simulink model "ES105A_StHlthSigNormn"  (R2013b)
settings: Solver=FixedStepDiscrete  SolverMode=SingleTasking  StartTime=0.0  StopTime=1  FixedStep=0.002  RelTol=1e-3
undefined symbols (not defined in the file): ARCHGLBPRM_FLOATZEROTHD_ULS_F32, CurrMeasCorrlnMaxErrCurr, CURRMOTSUMDIVBYZEROPROTNVAL_AMPR_F32, DIGTQDIVBYZEROPROTNVAL_HWNWTMTR_F32, DutyCycThermProtnDutyCycFildThd, EcuTMeasRngDiagcMax, EcuTMeasRngDiagcMin, EotLrngAuthyStrtLrn, FRICESTIMNDIVBYZEROPROTNVAL_HWNWTMTR_F32, HLTH0PERC_CNT_U08, HLTH100PERC_CNT_F32, HLTH100PERC_CNT_U08, HLTH50PERC_CNT_U08, HwTqCorrlnChATraSumSetFltThd, HwTqCorrlnChBTraSumSetFltThd, HWTQIDPTSIG_CNT_U08, MOTAG2MEAS_VALMAXERR_VOLTSQD_F32, MOTAG2MEAS_VALMINERR_VOLTSQD_F32, MOTAGCORRLN_MOTAGCORRLNERRTHD_MOTREVELEC_U0P16, MotDrvDiagcErrThd, MOTPOS2DIVBYZEROPROTNVAL2_VOLTSQD_F32, MOTPOS2DIVBYZEROPROTNVAL_VOLTSQD_F32, MOTPOSNERRDIVBYZEROPROTNVAL_MOTREV_U16, MOTPOSNERRZEROTHD_MOTREV_U0P16, NtcNr1, NtcSts1, PHAVLTGDIVBYZEROPROTNVAL_NANOSEC_F32, SigQlfr1, STHLTHSCAGFAC_CNT_F32, StHlthSigNormnAbsltMotPosDifStHlthDiagThd, StHlthSigNormnCurrMotSumStHlthDiagThd, StHlthSigNormnDigTqStHlthDiagThd, StHlthSigNormnDutyCycFltLimThd, StHlthSigNormnHiCtrlrT, StHlthSigNormnIdptSigStHlthSca, StHlthSigNormnLoCtrlrT, StHlthSigNormnMaxFricThd, StHlthSigNormnMinRackTrvlLim, StHlthSigNormnMotPosStHlthDiagThd, StHlthSigNormnMotVelCal, StHlthSigNormnPhaInfoStHlthDiagThd, StHlthSigNormnStHlthCorrlnErr, StHlthSigNormnStHlthCurrMotSum, StHlthSigNormnStHlthPhaInfo, StHlthSigNormnValMaxStHlthErr, StHlthSigNormnValMinStHlthErr, StHlthSigNormnWhlImbRejctnThd, SysGlbPrmMotPoleCnt, TSTHLTH0PERC_CNT_U08, u2, u3, u4, VLTGSTHLTH0PERC_CNT_U08
libraries: NxtrLim x39, simulink x33, NxtrAbslt x4
(part 4 of 10)

== system ES105A_StHlthSigNormn/StHlthSigNormn/UpdRawSig/Controller temperature/CtrlrTStHlth0Perc ==
  Action Port : ActionPort  ActionType=elseif
  Bitwise Operator : simulink/Logic and Bit Operations/Bitwise Operator  logicop=OR  UseBitMask=off  NumInputPorts=2  BitMask=bin2dec('11011001')  BitMaskRealWorld=Stored Integer
  Constant : Constant  Value=HLTH0PERC_CNT_U08  OutDataTypeStr=uint8
      settings: AttributesFormatString=%<OutDataTypeStr>
  Constant1 : Constant  OutDataTypeStr=uint8
      settings: AttributesFormatString=%<OutDataTypeStr>
  Constant2 : Constant  OutDataTypeStr=uint8
      settings: AttributesFormatString=%<OutDataTypeStr>
  CopyRight2 : Subsystem  Description=|  mask(Copyright Information){none=on}
      | Copyright info block.                                               
      |                                                                     
      | Place copyright information at the top of every subsystem in design.
      mask prompts: none "No parameters"
      mask help: Place copyright information at the top of every subsystem in design.
      mask Display:
      | NxtrConf = 'Nexteer Confidential';
      | 
      | sys = bdroot; %handle for the current model ("system")
      | first = get_param(sys,'Created');
      | first = first(end-3:end);  %year is last four digits
      | 
      | last = get_param(sys,'LastModifiedDate');
      | if isempty(last)
      |     last = datestr(now,'yyyy');
      | else
      |     last = last(end-3:end);
      | end
      | 
      | if strcmp(first,last)
      |     fprintf('%s -- Copyright %s Nexteer',NxtrConf,first)
      | else
      |     fprintf('%s -- %s%s- %s Nexteer',NxtrConf,char(169),first,last)
      | end
  Data Store Read : DataStoreRead  DataStoreName=EcuTRngIgnCyc
  Data Store Write : DataStoreWrite  DataStoreName=EcuTRngIgnCyc
  Shift Arithmetic : ArithShift  BitShiftNumber=LOTSTHLTH0PERC_CNT_U08  BitShiftDirection=Left
  Shift Arithmetic1 : ArithShift  BitShiftNumber=LOTSTHLTH0PERC_CNT_U08  BitShiftDirection=Left
  CtrlrTStHlth : Outport
  PrsntCtrlrTRng : Outport  Port=2
  wires:
  Shift Arithmetic1/1 -> PrsntCtrlrTRng/1
  Constant2/1 -> Shift Arithmetic1/1
  Bitwise Operator/1 -> Data Store Write/1
  Data Store Read/1 -> Bitwise Operator/1
  Shift Arithmetic/1 -> Bitwise Operator/2
  Constant1/1 -> Shift Arithmetic/1
  Constant/1 -> CtrlrTStHlth/1

== system ES105A_StHlthSigNormn/StHlthSigNormn/UpdRawSig/Controller temperature/CtrlrTStHlth0Perc1 ==
  Action Port : ActionPort  ActionType=else
  Bitwise Operator : simulink/Logic and Bit Operations/Bitwise Operator  logicop=OR  UseBitMask=off  NumInputPorts=2  BitMask=bin2dec('11011001')  BitMaskRealWorld=Stored Integer
  Constant : Constant  Value=HLTH0PERC_CNT_U08  OutDataTypeStr=uint8
      settings: AttributesFormatString=%<OutDataTypeStr>
  Constant1 : Constant  OutDataTypeStr=uint8
      settings: AttributesFormatString=%<OutDataTypeStr>
  Constant2 : Constant  OutDataTypeStr=uint8
      settings: AttributesFormatString=%<OutDataTypeStr>
  CopyRight2 : Subsystem  Description=|  mask(Copyright Information){none=on}
      | Copyright info block.                                               
      |                                                                     
      | Place copyright information at the top of every subsystem in design.
      mask prompts: none "No parameters"
      mask help: Place copyright information at the top of every subsystem in design.
      mask Display:
      | NxtrConf = 'Nexteer Confidential';
      | 
      | sys = bdroot; %handle for the current model ("system")
      | first = get_param(sys,'Created');
      | first = first(end-3:end);  %year is last four digits
      | 
      | last = get_param(sys,'LastModifiedDate');
      | if isempty(last)
      |     last = datestr(now,'yyyy');
      | else
      |     last = last(end-3:end);
      | end
      | 
      | if strcmp(first,last)
      |     fprintf('%s -- Copyright %s Nexteer',NxtrConf,first)
      | else
      |     fprintf('%s -- %s%s- %s Nexteer',NxtrConf,char(169),first,last)
      | end
  Data Store Read : DataStoreRead  DataStoreName=EcuTRngIgnCyc
  Data Store Write : DataStoreWrite  DataStoreName=EcuTRngIgnCyc
  Shift Arithmetic : ArithShift  BitShiftNumber=HITSTHLTH0PERC_CNT_U08  BitShiftDirection=Left
  Shift Arithmetic1 : ArithShift  BitShiftNumber=HITSTHLTH0PERC_CNT_U08  BitShiftDirection=Left
  CtrlrTStHlth : Outport
  PrsntCtrlrTRng : Outport  Port=2
  wires:
  Constant/1 -> CtrlrTStHlth/1
  Constant1/1 -> Shift Arithmetic/1
  Shift Arithmetic/1 -> Bitwise Operator/2
  Data Store Read/1 -> Bitwise Operator/1
  Bitwise Operator/1 -> Data Store Write/1
  Constant2/1 -> Shift Arithmetic1/1
  Shift Arithmetic1/1 -> PrsntCtrlrTRng/1

== system ES105A_StHlthSigNormn/StHlthSigNormn/UpdRawSig/Controller temperature/CtrlrTStHlth100Perc ==
  Action Port : ActionPort  ActionType=then
  Constant : Constant  Value=HLTH100PERC_CNT_U08  OutDataTypeStr=uint8
  Constant1 : Constant  Value=0  OutDataTypeStr=uint8
      settings: AttributesFormatString=%<OutDataTypeStr>
  CopyRight2 : Subsystem  Description=|  mask(Copyright Information){none=on}
      | Copyright info block.                                               
      |                                                                     
      | Place copyright information at the top of every subsystem in design.
      mask prompts: none "No parameters"
      mask help: Place copyright information at the top of every subsystem in design.
      mask Display:
      | NxtrConf = 'Nexteer Confidential';
      | 
      | sys = bdroot; %handle for the current model ("system")
      | first = get_param(sys,'Created');
      | first = first(end-3:end);  %year is last four digits
      | 
      | last = get_param(sys,'LastModifiedDate');
      | if isempty(last)
      |     last = datestr(now,'yyyy');
      | else
      |     last = last(end-3:end);
      | end
      | 
      | if strcmp(first,last)
      |     fprintf('%s -- Copyright %s Nexteer',NxtrConf,first)
      | else
      |     fprintf('%s -- %s%s- %s Nexteer',NxtrConf,char(169),first,last)
      | end
  CtrlrTStHlth : Outport
  PrsntCtrlrTRng : Outport  Port=2  InitialOutput=[0]
  wires:
  Constant/1 -> CtrlrTStHlth/1
  Constant1/1 -> PrsntCtrlrTRng/1

== system ES105A_StHlthSigNormn/StHlthSigNormn/UpdRawSig/Controller temperature/CtrlrTStHlth50Perc ==
  Action Port : ActionPort  ActionType=elseif
  Bitwise Operator : simulink/Logic and Bit Operations/Bitwise Operator  logicop=OR  UseBitMask=off  NumInputPorts=2  BitMask=bin2dec('11011001')  BitMaskRealWorld=Stored Integer
  Constant : Constant  Value=HLTH50PERC_CNT_U08  OutDataTypeStr=uint8
  Constant1 : Constant  OutDataTypeStr=uint8
      settings: AttributesFormatString=%<OutDataTypeStr>
  Constant2 : Constant  OutDataTypeStr=uint8
      settings: AttributesFormatString=%<OutDataTypeStr>
  CopyRight2 : Subsystem  Description=|  mask(Copyright Information){none=on}
      | Copyright info block.                                               
      |                                                                     
      | Place copyright information at the top of every subsystem in design.
      mask prompts: none "No parameters"
      mask help: Place copyright information at the top of every subsystem in design.
      mask Display:
      | NxtrConf = 'Nexteer Confidential';
      | 
      | sys = bdroot; %handle for the current model ("system")
      | first = get_param(sys,'Created');
      | first = first(end-3:end);  %year is last four digits
      | 
      | last = get_param(sys,'LastModifiedDate');
      | if isempty(last)
      |     last = datestr(now,'yyyy');
      | else
      |     last = last(end-3:end);
      | end
      | 
      | if strcmp(first,last)
      |     fprintf('%s -- Copyright %s Nexteer',NxtrConf,first)
      | else
      |     fprintf('%s -- %s%s- %s Nexteer',NxtrConf,char(169),first,last)
      | end
  Data Store Read : DataStoreRead  DataStoreName=EcuTRngIgnCyc
  Data Store Write : DataStoreWrite  DataStoreName=EcuTRngIgnCyc
  Shift Arithmetic : ArithShift  BitShiftNumber=LOTSTHLTH50PERC_CNT_U08  BitShiftDirection=Left
  Shift Arithmetic1 : ArithShift  BitShiftNumber=LOTSTHLTH50PERC_CNT_U08  BitShiftDirection=Left
  CtrlrTStHlth : Outport
  PrsntCtrlrTRng : Outport  Port=2
  wires:
  Constant/1 -> CtrlrTStHlth/1
  Constant1/1 -> Shift Arithmetic/1
  Shift Arithmetic/1 -> Bitwise Operator/2
  Data Store Read/1 -> Bitwise Operator/1
  Bitwise Operator/1 -> Data Store Write/1
  Constant2/1 -> Shift Arithmetic1/1
  Shift Arithmetic1/1 -> PrsntCtrlrTRng/1

== system ES105A_StHlthSigNormn/StHlthSigNormn/UpdRawSig/Controller temperature/CtrlrTStHlth50Perc1 ==
  Action Port : ActionPort  ActionType=elseif
  Bitwise Operator : simulink/Logic and Bit Operations/Bitwise Operator  logicop=OR  UseBitMask=off  NumInputPorts=2  BitMask=bin2dec('11011001')  BitMaskRealWorld=Stored Integer
  Constant : Constant  Value=HLTH50PERC_CNT_U08  OutDataTypeStr=uint8
      settings: AttributesFormatString=%<OutDataTypeStr>
  Constant1 : Constant  OutDataTypeStr=uint8
      settings: AttributesFormatString=%<OutDataTypeStr>
  Constant2 : Constant  OutDataTypeStr=uint8
      settings: AttributesFormatString=%<OutDataTypeStr>
  CopyRight2 : Subsystem  Description=|  mask(Copyright Information){none=on}
      | Copyright info block.                                               
      |                                                                     
      | Place copyright information at the top of every subsystem in design.
      mask prompts: none "No parameters"
      mask help: Place copyright information at the top of every subsystem in design.
      mask Display:
      | NxtrConf = 'Nexteer Confidential';
      | 
      | sys = bdroot; %handle for the current model ("system")
      | first = get_param(sys,'Created');
      | first = first(end-3:end);  %year is last four digits
      | 
      | last = get_param(sys,'LastModifiedDate');
      | if isempty(last)
      |     last = datestr(now,'yyyy');
      | else
      |     last = last(end-3:end);
      | end
      | 
      | if strcmp(first,last)
      |     fprintf('%s -- Copyright %s Nexteer',NxtrConf,first)
      | else
      |     fprintf('%s -- %s%s- %s Nexteer',NxtrConf,char(169),first,last)
      | end
  Data Store Read : DataStoreRead  DataStoreName=EcuTRngIgnCyc
  Data Store Write : DataStoreWrite  DataStoreName=EcuTRngIgnCyc
  Shift Arithmetic : ArithShift  BitShiftNumber=HITSTHLTH50PERC_CNT_U08  BitShiftDirection=Left
  Shift Arithmetic1 : ArithShift  BitShiftNumber=HITSTHLTH50PERC_CNT_U08  BitShiftDirection=Left
  CtrlrTStHlth : Outport
  PrsntCtrlrTRng : Outport  Port=2
  wires:
  Constant/1 -> CtrlrTStHlth/1
  Constant1/1 -> Shift Arithmetic/1
  Shift Arithmetic/1 -> Bitwise Operator/2
  Data Store Read/1 -> Bitwise Operator/1
  Bitwise Operator/1 -> Data Store Write/1
  Constant2/1 -> Shift Arithmetic1/1
  Shift Arithmetic1/1 -> PrsntCtrlrTRng/1

== system ES105A_StHlthSigNormn/StHlthSigNormn/UpdRawSig/Current Error/CopyRight2 ==

== system ES105A_StHlthSigNormn/StHlthSigNormn/UpdRawSig/Current Error/CurrMotSumABCStHlth Calc ==
  CurrMotSumABC : Inport
  Action Port : ActionPort  ActionType=case
  Constant : Constant  Value=StHlthSigNormnStHlthCurrMotSum
  CopyRight2 : Subsystem  Description=|  mask(Copyright Information){none=on}
      | Copyright info block.                                               
      |                                                                     
      | Place copyright information at the top of every subsystem in design.
      mask prompts: none "No parameters"
      mask help: Place copyright information at the top of every subsystem in design.
      mask Display:
      | NxtrConf = 'Nexteer Confidential';
      | 
      | sys = bdroot; %handle for the current model ("system")
      | first = get_param(sys,'Created');
      | first = first(end-3:end);  %year is last four digits
      | 
      | last = get_param(sys,'LastModifiedDate');
      | if isempty(last)
      |     last = datestr(now,'yyyy');
      | else
      |     last = last(end-3:end);
      | end
      | 
      | if strcmp(first,last)
      |     fprintf('%s -- Copyright %s Nexteer',NxtrConf,first)
      | else
      |     fprintf('%s -- %s%s- %s Nexteer',NxtrConf,char(169),first,last)
      | end
  If : If  IfExpression=u1
  If Action Subsystem : Subsystem  TreatAsAtomicUnit=on
  If Action Subsystem1 : Subsystem  TreatAsAtomicUnit=on
  LimStat_u2 : NxtrLim/LimStat_u08  LoLim=CurrMotSumABCStHlth.EngMin  HiLim=CurrMotSumABCStHlth.EngMax
      settings: AttributesFormatString=|
      | Low Limit: %<LoLim>
      | High Limit:%<HiLim>
  Merge : Merge
  Relational Operator : RelationalOperator  Operator=>  OutDataTypeStr=boolean
  CurrMotSumABCStHlth : Outport  InitialOutput=HLTH100PERC_CNT_U08
      settings: AttributesFormatString=Initial Output: %<InitialOutput>
  wires:
  CurrMotSumABC/1 -> [CurrMotSumABC], Relational Operator/1
  Constant/1 -> Relational Operator/2
  Relational Operator/1 -> If/1
  If/1 -> If Action Subsystem/Action
  If/2 -> If Action Subsystem1/Action
  [CurrMotSumABC] -> If Action Subsystem/1(CurrMotSumABC)
  If Action Subsystem/1(CurrMotSumABCStHlth) -> Merge/1
  If Action Subsystem1/1(CurrMotSumABCStHlth) -> Merge/2
  Merge/1 -> LimStat_u2/1
  LimStat_u2/1 -> CurrMotSumABCStHlth/1

== system ES105A_StHlthSigNormn/StHlthSigNormn/UpdRawSig/Current Error/CurrMotSumDEFStHlth Calc ==
  CurrMotSumDEF : Inport
  Action Port : ActionPort  ActionType=default
  Constant2 : Constant  Value=StHlthSigNormnStHlthCurrMotSum
  CopyRight2 : Subsystem  Description=|  mask(Copyright Information){none=on}
      | Copyright info block.                                               
      |                                                                     
      | Place copyright information at the top of every subsystem in design.
      mask prompts: none "No parameters"
      mask help: Place copyright information at the top of every subsystem in design.
      mask Display:
      | NxtrConf = 'Nexteer Confidential';
      | 
      | sys = bdroot; %handle for the current model ("system")
      | first = get_param(sys,'Created');
      | first = first(end-3:end);  %year is last four digits
      | 
      | last = get_param(sys,'LastModifiedDate');
      | if isempty(last)
      |     last = datestr(now,'yyyy');
      | else
      |     last = last(end-3:end);
      | end
      | 
      | if strcmp(first,last)
      |     fprintf('%s -- Copyright %s Nexteer',NxtrConf,first)
      | else
      |     fprintf('%s -- %s%s- %s Nexteer',NxtrConf,char(169),first,last)
      | end
  If Action Subsystem4 : Subsystem  TreatAsAtomicUnit=on
  If Action Subsystem5 : Subsystem  TreatAsAtomicUnit=on
  If2 : If  IfExpression=u1
  LimStat_u1 : NxtrLim/LimStat_u08  LoLim=CurrMotSumDEFStHlth.EngMin  HiLim=CurrMotSumDEFStHlth.EngMax
      settings: AttributesFormatString=|
      | Low Limit: %<LoLim>
      | High Limit:%<HiLim>
  Merge1 : Merge
  Relational Operator2 : RelationalOperator  Operator=>  OutDataTypeStr=boolean
  CurrMotSumDEFStHlth : Outport  InitialOutput=HLTH100PERC_CNT_U08
      settings: AttributesFormatString=Initial Output: %<InitialOutput>
  wires:
  CurrMotSumDEF/1 -> [CurrMotSumDEF], Relational Operator2/1
  Constant2/1 -> Relational Operator2/2
  Relational Operator2/1 -> If2/1
  If2/1 -> If Action Subsystem4/Action
  If2/2 -> If Action Subsystem5/Action
  [CurrMotSumDEF] -> If Action Subsystem4/1(CurrMotSumDEF)
  If Action Subsystem4/1(CurrMotSumDEFStHlth) -> Merge1/1
  If Action Subsystem5/1(CurrMotSumDEFStHlth) -> Merge1/2
  Merge1/1 -> LimStat_u1/1
  LimStat_u1/1 -> CurrMotSumDEFStHlth/1

== system ES105A_StHlthSigNormn/StHlthSigNormn/UpdRawSig/Current Error/CurrMotSumPhaStHlth ==
  NtcNr : Inport
  NtcStInfo : Inport  Port=2
  NtcSts : Inport  Port=3
  DebStep : Inport  Port=4
  SetNtcSts : Subsystem  RequirementInfo={} %GIDa_d68da11a_5186_43bd_ae15_b68d94f31a5a  TreatAsAtomicUnit=on
      settings: RTWSystemCode=Inline
  wires:
  NtcNr/1 -> SetNtcSts/1(NtcNr)  "NtcNr"
  NtcSts/1 -> SetNtcSts/3(NtcSts)
  DebStep/1 -> SetNtcSts/4(DebStep)
  NtcStInfo/1 -> SetNtcSts/2(NtcStInfo)

== system ES105A_StHlthSigNormn/StHlthSigNormn/UpdRawSig/Current Error/NTC Sts Calculation ==
  StHlthErr : Inport
  CopyRight2 : Subsystem  Description=|  mask(Copyright Information){none=on}
      | Copyright info block.                                               
      |                                                                     
      | Place copyright information at the top of every subsystem in design.
      mask prompts: none "No parameters"
      mask help: Place copyright information at the top of every subsystem in design.
      mask Display:
      | NxtrConf = 'Nexteer Confidential';
      | 
      | sys = bdroot; %handle for the current model ("system")
      | first = get_param(sys,'Created');
      | first = first(end-3:end);  %year is last four digits
      | 
      | last = get_param(sys,'LastModifiedDate');
      | if isempty(last)
      |     last = datestr(now,'yyyy');
      | else
      |     last = last(end-3:end);
      | end
      | 
      | if strcmp(first,last)
      |     fprintf('%s -- Copyright %s Nexteer',NxtrConf,first)
      | else
      |     fprintf('%s -- %s%s- %s Nexteer',NxtrConf,char(169),first,last)
      | end
  If : If  IfExpression=u1
  Merge : Merge
  NtcFaild : Subsystem  TreatAsAtomicUnit=on
  NtcPassd : Subsystem  TreatAsAtomicUnit=on
  NtcSts : Outport
  wires:
  StHlthErr/1 -> If/1
  If/1 -> NtcFaild/Action
  Merge/1 -> NtcSts/1
  NtcPassd/1(NtcPassd) -> Merge/2
  If/2 -> NtcPassd/Action
  NtcFaild/1(NtcFaild) -> Merge/1

== system ES105A_StHlthSigNormn/StHlthSigNormn/UpdRawSig/Default/CopyRight2 ==

== system ES105A_StHlthSigNormn/StHlthSigNormn/UpdRawSig/Digital Torque Sensor /CopyRight2 ==

== system ES105A_StHlthSigNormn/StHlthSigNormn/UpdRawSig/Digital Torque Sensor /DigTqIdptSigStHlth Calc ==
  HwTqIdptSig : Inport
  Action Port : ActionPort  ActionType=default
  Constant2 : Constant  Value=HWTQIDPTSIG_CNT_U08
  CopyRight2 : Subsystem  Description=|  mask(Copyright Information){none=on}
      | Copyright info block.                                               
      |                                                                     
      | Place copyright information at the top of every subsystem in design.
      mask prompts: none "No parameters"
      mask help: Place copyright information at the top of every subsystem in design.
      mask Display:
      | NxtrConf = 'Nexteer Confidential';
      | 
      | sys = bdroot; %handle for the current model ("system")
      | first = get_param(sys,'Created');
      | first = first(end-3:end);  %year is last four digits
      | 
      | last = get_param(sys,'LastModifiedDate');
      | if isempty(last)
      |     last = datestr(now,'yyyy');
      | else
      |     last = last(end-3:end);
      | end
      | 
      | if strcmp(first,last)
      |     fprintf('%s -- Copyright %s Nexteer',NxtrConf,first)
      | else
      |     fprintf('%s -- %s%s- %s Nexteer',NxtrConf,char(169),first,last)
      | end
  If Action Subsystem4 : Subsystem  TreatAsAtomicUnit=on
  If Action Subsystem5 : Subsystem  TreatAsAtomicUnit=on
  If2 : If  IfExpression=u1
  LimStat_u2 : NxtrLim/LimStat_u08  LoLim=DigTqIdptSigStHlth.EngMin  HiLim=DigTqIdptSigStHlth.EngMax
      settings: AttributesFormatString=|
      | Low Limit: %<LoLim>
      | High Limit:%<HiLim>
  Merge2 : Merge
  Relational Operator2 : RelationalOperator  Operator===  OutDataTypeStr=boolean
  " DigTqIdptSigStHlth" : Outport  InitialOutput=HLTH100PERC_CNT_U08
      settings: AttributesFormatString=Initial Output: %<InitialOutput>
  wires:
  Relational Operator2/1 -> If2/1
  If2/1 -> If Action Subsystem4/Action
  If2/2 -> If Action Subsystem5/Action
  HwTqIdptSig/1 -> If Action Subsystem5/1(HwTqIdptSig), Relational Operator2/1
  If Action Subsystem4/1(DigTqIdptSigStHlth) -> Merge2/1
  Merge2/1 -> LimStat_u2/1
  Constant2/1 -> Relational Operator2/2
  If Action Subsystem5/1(DigTqIdptSigStHlth) -> Merge2/2
  LimStat_u2/1 -> " DigTqIdptSigStHlth"/1

== system ES105A_StHlthSigNormn/StHlthSigNormn/UpdRawSig/Digital Torque Sensor /DigTqSnsrAStHlth Calc ==
  HwTqChACorrlnTraErr : Inport
  Action Port : ActionPort  ActionType=case
  Abslt_f32_f32 : NxtrAbslt/Abslt_f32_f32  SFunctionSpec=single y1 = Abslt_f32_f32(single u1)
      settings: AttributesFormatString=%<Name>
  Constant : Constant  Value=HwTqCorrlnChATraSumSetFltThd
  CopyRight2 : Subsystem  Description=|  mask(Copyright Information){none=on}
      | Copyright info block.                                               
      |                                                                     
      | Place copyright information at the top of every subsystem in design.
      mask prompts: none "No parameters"
      mask help: Place copyright information at the top of every subsystem in design.
      mask Display:
      | NxtrConf = 'Nexteer Confidential';
      | 
      | sys = bdroot; %handle for the current model ("system")
      | first = get_param(sys,'Created');
      | first = first(end-3:end);  %year is last four digits
      | 
      | last = get_param(sys,'LastModifiedDate');
      | if isempty(last)
      |     last = datestr(now,'yyyy');
      | else
      |     last = last(end-3:end);
      | end
      | 
      | if strcmp(first,last)
      |     fprintf('%s -- Copyright %s Nexteer',NxtrConf,first)
      | else
      |     fprintf('%s -- %s%s- %s Nexteer',NxtrConf,char(169),first,last)
      | end
  If : If  IfExpression=u1
  If Action Subsystem : Subsystem  TreatAsAtomicUnit=on
  If Action Subsystem1 : Subsystem  TreatAsAtomicUnit=on
  LimStat_u08 : NxtrLim/LimStat_u08  LoLim=DigTqSnsrAStHlth.EngMin  HiLim=DigTqSnsrAStHlth.EngMax
      settings: AttributesFormatString=|
      | Low Limit: %<LoLim>
      | High Limit:%<HiLim>
  Merge : Merge
  Relational Operator : RelationalOperator  Operator=>  OutDataTypeStr=boolean
  DigTqSnsrAStHlth : Outport  InitialOutput=HLTH100PERC_CNT_U08
      settings: AttributesFormatString=Initial Output: %<InitialOutput>
  wires:
  Merge/1 -> LimStat_u08/1
  Abslt_f32_f32/1 -> Relational Operator/1
  Constant/1 -> Relational Operator/2
  Relational Operator/1 -> If/1
  If/1 -> If Action Subsystem/Action
  If/2 -> If Action Subsystem1/Action
  HwTqChACorrlnTraErr/1 -> Abslt_f32_f32/1, If Action Subsystem1/1(HwTqChACorrlnTraErr)
  If Action Subsystem/1(DigTqSnsrAStHlth) -> Merge/1
  If Action Subsystem1/1(DigTqSnsrAStHlth) -> Merge/2
  LimStat_u08/1 -> DigTqSnsrAStHlth/1

== system ES105A_StHlthSigNormn/StHlthSigNormn/UpdRawSig/Digital Torque Sensor /DigTqSnsrBStHlth Calc ==
  HwTqChBCorrlnTraErr : Inport
  Action Port : ActionPort  ActionType=case
  Abslt_f32_f1 : NxtrAbslt/Abslt_f32_f32  SFunctionSpec=single y1 = Abslt_f32_f32(single u1)
      settings: AttributesFormatString=%<Name>
  Constant1 : Constant  Value=HwTqCorrlnChBTraSumSetFltThd
  CopyRight2 : Subsystem  Description=|  mask(Copyright Information){none=on}
      | Copyright info block.                                               
      |                                                                     
      | Place copyright information at the top of every subsystem in design.
      mask prompts: none "No parameters"
      mask help: Place copyright information at the top of every subsystem in design.
      mask Display:
      | NxtrConf = 'Nexteer Confidential';
      | 
      | sys = bdroot; %handle for the current model ("system")
      | first = get_param(sys,'Created');
      | first = first(end-3:end);  %year is last four digits
      | 
      | last = get_param(sys,'LastModifiedDate');
      | if isempty(last)
      |     last = datestr(now,'yyyy');
      | else
      |     last = last(end-3:end);
      | end
      | 
      | if strcmp(first,last)
      |     fprintf('%s -- Copyright %s Nexteer',NxtrConf,first)
      | else
      |     fprintf('%s -- %s%s- %s Nexteer',NxtrConf,char(169),first,last)
      | end
  If Action Subsystem2 : Subsystem  TreatAsAtomicUnit=on
  If Action Subsystem3 : Subsystem  TreatAsAtomicUnit=on
  If1 : If  IfExpression=u1
  LimStat_u1 : NxtrLim/LimStat_u08  LoLim=DigTqSnsrBStHlth.EngMin  HiLim=DigTqSnsrBStHlth.EngMax
      settings: AttributesFormatString=|
      | Low Limit: %<LoLim>
      | High Limit:%<HiLim>
  Merge1 : Merge
  Relational Operator1 : RelationalOperator  Operator=>  OutDataTypeStr=boolean
  DigTqSnsrBStHlth : Outport  InitialOutput=HLTH100PERC_CNT_U08
      settings: AttributesFormatString=Initial Output: %<InitialOutput>
  wires:
  Merge1/1 -> LimStat_u1/1
  Abslt_f32_f1/1 -> Relational Operator1/1
  Constant1/1 -> Relational Operator1/2
  Relational Operator1/1 -> If1/1
  If1/1 -> If Action Subsystem2/Action
  If1/2 -> If Action Subsystem3/Action
  HwTqChBCorrlnTraErr/1 -> Abslt_f32_f1/1, If Action Subsystem3/1(HwTqChBCorrlnTraErr)
  If Action Subsystem2/1(DigTqSnsrBStHlth) -> Merge1/1
  If Action Subsystem3/1(DigTqSnsrBStHlth) -> Merge1/2
  LimStat_u1/1 -> DigTqSnsrBStHlth/1

== system ES105A_StHlthSigNormn/StHlthSigNormn/UpdRawSig/Digital Torque Sensor /DigTqSnsrPhaStHlth ==
  NtcNr : Inport
  NtcStInfo : Inport  Port=2
  NtcSts : Inport  Port=3
  DebStep : Inport  Port=4
  SetNtcSts : Subsystem  RequirementInfo={} %GIDa_2e8106b4_b705_4f70_a166_c375d4b30e66  TreatAsAtomicUnit=on
      settings: RTWSystemCode=Inline
  wires:
  NtcNr/1 -> SetNtcSts/1(NtcNr)  "NtcNr"
  NtcSts/1 -> SetNtcSts/3(NtcSts)
  DebStep/1 -> SetNtcSts/4(DebStep)
  NtcStInfo/1 -> SetNtcSts/2(NtcStInfo)

== system ES105A_StHlthSigNormn/StHlthSigNormn/UpdRawSig/Digital Torque Sensor /NTC Sts Calculation ==
  StHlthErr : Inport
  CopyRight2 : Subsystem  Description=|  mask(Copyright Information){none=on}
      | Copyright info block.                                               
      |                                                                     
      | Place copyright information at the top of every subsystem in design.
      mask prompts: none "No parameters"
      mask help: Place copyright information at the top of every subsystem in design.
      mask Display:
      | NxtrConf = 'Nexteer Confidential';
      | 
      | sys = bdroot; %handle for the current model ("system")
      | first = get_param(sys,'Created');
      | first = first(end-3:end);  %year is last four digits
      | 
      | last = get_param(sys,'LastModifiedDate');
      | if isempty(last)
      |     last = datestr(now,'yyyy');
      | else
      |     last = last(end-3:end);
      | end
      | 
      | if strcmp(first,last)
      |     fprintf('%s -- Copyright %s Nexteer',NxtrConf,first)
      | else
      |     fprintf('%s -- %s%s- %s Nexteer',NxtrConf,char(169),first,last)
      | end
  If : If  IfExpression=u1
  Merge : Merge
  NtcFaild : Subsystem  TreatAsAtomicUnit=on
  NtcPassd : Subsystem  TreatAsAtomicUnit=on
  NtcSts : Outport
  wires:
  StHlthErr/1 -> If/1
  If/1 -> NtcFaild/Action
  Merge/1 -> NtcSts/1
  NtcPassd/1(NtcPassd) -> Merge/2
  If/2 -> NtcPassd/Action
  NtcFaild/1(NtcFaild) -> Merge/1

== system ES105A_StHlthSigNormn/StHlthSigNormn/UpdRawSig/Duty Cycle Exceeded/CopyRight2 ==

== system ES105A_StHlthSigNormn/StHlthSigNormn/UpdRawSig/Duty Cycle Exceeded/If Action Subsystem ==
  Action Port : ActionPort  ActionType=then
  Constant : Constant  Value=HLTH0PERC_CNT_U08
  CopyRight2 : Subsystem  Description=|  mask(Copyright Information){none=on}
      | Copyright info block.                                               
      |                                                                     
      | Place copyright information at the top of every subsystem in design.
      mask prompts: none "No parameters"
      mask help: Place copyright information at the top of every subsystem in design.
      mask Display:
      | NxtrConf = 'Nexteer Confidential';
      | 
      | sys = bdroot; %handle for the current model ("system")
      | first = get_param(sys,'Created');
      | first = first(end-3:end);  %year is last four digits
      | 
      | last = get_param(sys,'LastModifiedDate');
      | if isempty(last)
      |     last = datestr(now,'yyyy');
      | else
      |     last = last(end-3:end);
      | end
      | 
      | if strcmp(first,last)
      |     fprintf('%s -- Copyright %s Nexteer',NxtrConf,first)
      | else
      |     fprintf('%s -- %s%s- %s Nexteer',NxtrConf,char(169),first,last)
      | end
  DutyCycStHlth : Outport
  wires:
  Constant/1 -> DutyCycStHlth/1

== system ES105A_StHlthSigNormn/StHlthSigNormn/UpdRawSig/Duty Cycle Exceeded/If Action Subsystem1 ==
  Action Port : ActionPort  ActionType=elseif
  Constant : Constant  Value=HLTH50PERC_CNT_U08
  CopyRight2 : Subsystem  Description=|  mask(Copyright Information){none=on}
      | Copyright info block.                                               
      |                                                                     
      | Place copyright information at the top of every subsystem in design.
      mask prompts: none "No parameters"
      mask help: Place copyright information at the top of every subsystem in design.
      mask Display:
      | NxtrConf = 'Nexteer Confidential';
      | 
      | sys = bdroot; %handle for the current model ("system")
      | first = get_param(sys,'Created');
      | first = first(end-3:end);  %year is last four digits
      | 
      | last = get_param(sys,'LastModifiedDate');
      | if isempty(last)
      |     last = datestr(now,'yyyy');
      | else
      |     last = last(end-3:end);
      | end
      | 
      | if strcmp(first,last)
      |     fprintf('%s -- Copyright %s Nexteer',NxtrConf,first)
      | else
      |     fprintf('%s -- %s%s- %s Nexteer',NxtrConf,char(169),first,last)
      | end
  DutyCycStHlth : Outport
  wires:
  Constant/1 -> DutyCycStHlth/1

== system ES105A_StHlthSigNormn/StHlthSigNormn/UpdRawSig/Duty Cycle Exceeded/If Action Subsystem2 ==
  Action Port : ActionPort  ActionType=else
  Constant : Constant  Value=HLTH100PERC_CNT_U08
  CopyRight2 : Subsystem  Description=|  mask(Copyright Information){none=on}
      | Copyright info block.                                               
      |                                                                     
      | Place copyright information at the top of every subsystem in design.
      mask prompts: none "No parameters"
      mask help: Place copyright information at the top of every subsystem in design.
      mask Display:
      | NxtrConf = 'Nexteer Confidential';
      | 
      | sys = bdroot; %handle for the current model ("system")
      | first = get_param(sys,'Created');
      | first = first(end-3:end);  %year is last four digits
      | 
      | last = get_param(sys,'LastModifiedDate');
      | if isempty(last)
      |     last = datestr(now,'yyyy');
      | else
      |     last = last(end-3:end);
      | end
      | 
      | if strcmp(first,last)
      |     fprintf('%s -- Copyright %s Nexteer',NxtrConf,first)
      | else
      |     fprintf('%s -- %s%s- %s Nexteer',NxtrConf,char(169),first,last)
      | end
  DutyCycStHlth : Outport
  wires:
  Constant/1 -> DutyCycStHlth/1

== system ES105A_StHlthSigNormn/StHlthSigNormn/UpdRawSig/Friction Estimation/CopyRight2 ==

== system ES105A_StHlthSigNormn/StHlthSigNormn/UpdRawSig/Friction Estimation/If Action Subsystem3 ==
  Action Port : ActionPort  ActionType=else
  Constant : Constant  Value=HLTH0PERC_CNT_U08
  CopyRight2 : Subsystem  Description=|  mask(Copyright Information){none=on}
      | Copyright info block.                                               
      |                                                                     
      | Place copyright information at the top of every subsystem in design.
      mask prompts: none "No parameters"
      mask help: Place copyright information at the top of every subsystem in design.
      mask Display:
      | NxtrConf = 'Nexteer Confidential';
      | 
      | sys = bdroot; %handle for the current model ("system")
      | first = get_param(sys,'Created');
      | first = first(end-3:end);  %year is last four digits
      | 
      | last = get_param(sys,'LastModifiedDate');
      | if isempty(last)
      |     last = datestr(now,'yyyy');
      | else
      |     last = last(end-3:end);
      | end
      | 
      | if strcmp(first,last)
      |     fprintf('%s -- Copyright %s Nexteer',NxtrConf,first)
      | else
      |     fprintf('%s -- %s%s- %s Nexteer',NxtrConf,char(169),first,last)
      | end
  FricEstStHlth : Outport
  wires:
  Constant/1 -> FricEstStHlth/1

== system ES105A_StHlthSigNormn/StHlthSigNormn/UpdRawSig/Friction Estimation/If Action Subsystem4 ==
  MaxLrndFric : Inport
  EOLFric : Inport  Port=2
  Action Port : ActionPort  ActionType=then
  Abs : Abs
  Add : Sum  Inputs=+-
  Add1 : Sum  Inputs=+-
  Constant1 : Constant  OutDataTypeStr=single
      settings: AttributesFormatString=%<OutDataTypeStr>
  Constant4 : Constant  Value=HLTH100PERC_CNT_F32
  CopyRight2 : Subsystem  Description=|  mask(Copyright Information){none=on}
      | Copyright info block.                                               
      |                                                                     
      | Place copyright information at the top of every subsystem in design.
      mask prompts: none "No parameters"
      mask help: Place copyright information at the top of every subsystem in design.
      mask Display:
      | NxtrConf = 'Nexteer Confidential';
      | 
      | sys = bdroot; %handle for the current model ("system")
      | first = get_param(sys,'Created');
      | first = first(end-3:end);  %year is last four digits
      | 
      | last = get_param(sys,'LastModifiedDate');
      | if isempty(last)
      |     last = datestr(now,'yyyy');
      | else
      |     last = last(end-3:end);
      | end
      | 
      | if strcmp(first,last)
      |     fprintf('%s -- Copyright %s Nexteer',NxtrConf,first)
      | else
      |     fprintf('%s -- %s%s- %s Nexteer',NxtrConf,char(169),first,last)
      | end
  Data Type Conversion : DataTypeConversion  OutDataTypeStr=uint8
  Divide : Product  Inputs=*/
  Divide by Zero Protection for Cal : Subsystem
  LimStat_f32 : NxtrLim/LimStat_f32  LoLim=FRICESTSTHLTHLOLI_CNT_F32  HiLim=FRICESTSTHLTHHILI_CNT_F32
      settings: AttributesFormatString=|
      | Low Limit: %<LoLim>
      | High Limit:%<HiLim>
  Product : Product
  FricEstStHlth : Outport
  wires:
  Constant1/1 -> Add/1
  Constant4/1 -> Product/2
  LimStat_f32/1 -> Data Type Conversion/1
  Data Type Conversion/1 -> FricEstStHlth/1
  Divide by Zero Protection for Cal/1(FricEstDelta) -> Divide/2
  MaxLrndFric/1 -> Add1/1
  Product/1 -> LimStat_f32/1
  Add/1 -> Product/1
  EOLFric/1 -> Add1/2, [EOLFric]
  Divide/1 -> Add/2
  Add1/1 -> Abs/1
  Abs/1 -> Divide/1
  [EOLFric] -> Divide by Zero Protection for Cal/1(EOLFric)

== system ES105A_StHlthSigNormn/StHlthSigNormn/UpdRawSig/Motor Position 2 /CopyRight2 ==

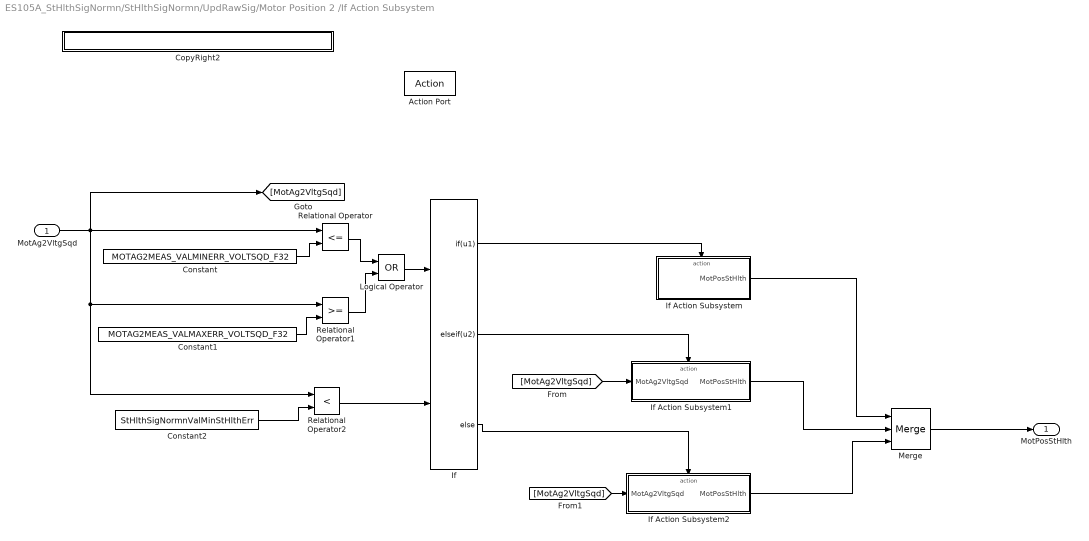
== system ES105A_StHlthSigNormn/StHlthSigNormn/UpdRawSig/Motor Position 2 /If Action Subsystem ==
  MotAg2VltgSqd : Inport
  Action Port : ActionPort  ActionType=then
  Constant : Constant  Value=MOTAG2MEAS_VALMINERR_VOLTSQD_F32
  Constant1 : Constant  Value=MOTAG2MEAS_VALMAXERR_VOLTSQD_F32
  Constant2 : Constant  Value=StHlthSigNormnValMinStHlthErr
  CopyRight2 : Subsystem  Description=|  mask(Copyright Information){none=on}
      | Copyright info block.                                               
      |                                                                     
      | Place copyright information at the top of every subsystem in design.
      mask prompts: none "No parameters"
      mask help: Place copyright information at the top of every subsystem in design.
      mask Display:
      | NxtrConf = 'Nexteer Confidential';
      | 
      | sys = bdroot; %handle for the current model ("system")
      | first = get_param(sys,'Created');
      | first = first(end-3:end);  %year is last four digits
      | 
      | last = get_param(sys,'LastModifiedDate');
      | if isempty(last)
      |     last = datestr(now,'yyyy');
      | else
      |     last = last(end-3:end);
      | end
      | 
      | if strcmp(first,last)
      |     fprintf('%s -- Copyright %s Nexteer',NxtrConf,first)
      | else
      |     fprintf('%s -- %s%s- %s Nexteer',NxtrConf,char(169),first,last)
      | end
  If : If  NumInputs=2  IfExpression=u1  ElseIfExpressions=u2
  If Action Subsystem : Subsystem  TreatAsAtomicUnit=on
  If Action Subsystem1 : Subsystem  TreatAsAtomicUnit=on
  If Action Subsystem2 : Subsystem  TreatAsAtomicUnit=on
  Logical Operator : Logic  Operator=OR  AllPortsSameDT=off  OutDataTypeStr=boolean
  Merge : Merge  Inputs=3
  Relational Operator : RelationalOperator  Operator=<=  OutDataTypeStr=boolean
  Relational Operator1 : RelationalOperator  OutDataTypeStr=boolean
  Relational Operator2 : RelationalOperator  Operator=<  OutDataTypeStr=boolean
  MotPosStHlth : Outport
  wires:
  Constant/1 -> Relational Operator/2
  MotAg2VltgSqd/1 -> Relational Operator/1, [MotAg2VltgSqd], Relational Operator1/1, Relational Operator2/1
  Constant1/1 -> Relational Operator1/2
  Relational Operator/1 -> Logical Operator/1
  Relational Operator1/1 -> Logical Operator/2
  Logical Operator/1 -> If/1
  If/1 -> If Action Subsystem/Action
  Constant2/1 -> Relational Operator2/2
  Relational Operator2/1 -> If/2
  If/2 -> If Action Subsystem1/Action
  If/3 -> If Action Subsystem2/Action
  [MotAg2VltgSqd] -> If Action Subsystem1/1(MotAg2VltgSqd)
  [MotAg2VltgSqd] -> If Action Subsystem2/1(MotAg2VltgSqd)
  If Action Subsystem/1(MotPosStHlth) -> Merge/1
  Merge/1 -> MotPosStHlth/1
  If Action Subsystem2/1(MotPosStHlth) -> Merge/3
  If Action Subsystem1/1(MotPosStHlth) -> Merge/2

== system ES105A_StHlthSigNormn/StHlthSigNormn/UpdRawSig/Motor Position 2 /If Action Subsystem1 ==
  Action Port : ActionPort  ActionType=else
  Constant : Constant  Value=HLTH100PERC_CNT_U08
  CopyRight2 : Subsystem  Description=|  mask(Copyright Information){none=on}
      | Copyright info block.                                               
      |                                                                     
      | Place copyright information at the top of every subsystem in design.
      mask prompts: none "No parameters"
      mask help: Place copyright information at the top of every subsystem in design.
      mask Display:
      | NxtrConf = 'Nexteer Confidential';
      | 
      | sys = bdroot; %handle for the current model ("system")
      | first = get_param(sys,'Created');
      | first = first(end-3:end);  %year is last four digits
      | 
      | last = get_param(sys,'LastModifiedDate');
      | if isempty(last)
      |     last = datestr(now,'yyyy');
      | else
      |     last = last(end-3:end);
      | end
      | 
      | if strcmp(first,last)
      |     fprintf('%s -- Copyright %s Nexteer',NxtrConf,first)
      | else
      |     fprintf('%s -- %s%s- %s Nexteer',NxtrConf,char(169),first,last)
      | end
  MotPosStHlth : Outport
  wires:
  Constant/1 -> MotPosStHlth/1

== system ES105A_StHlthSigNormn/StHlthSigNormn/UpdRawSig/Motor Position 2 /NTC Sts Calculation ==
  StHlthErr : Inport
  CopyRight2 : Subsystem  Description=|  mask(Copyright Information){none=on}
      | Copyright info block.                                               
      |                                                                     
      | Place copyright information at the top of every subsystem in design.
      mask prompts: none "No parameters"
      mask help: Place copyright information at the top of every subsystem in design.
      mask Display:
      | NxtrConf = 'Nexteer Confidential';
      | 
      | sys = bdroot; %handle for the current model ("system")
      | first = get_param(sys,'Created');
      | first = first(end-3:end);  %year is last four digits
      | 
      | last = get_param(sys,'LastModifiedDate');
      | if isempty(last)
      |     last = datestr(now,'yyyy');
      | else
      |     last = last(end-3:end);
      | end
      | 
      | if strcmp(first,last)
      |     fprintf('%s -- Copyright %s Nexteer',NxtrConf,first)
      | else
      |     fprintf('%s -- %s%s- %s Nexteer',NxtrConf,char(169),first,last)
      | end
  If : If  IfExpression=u1
  Merge : Merge
  NtcFaild : Subsystem  TreatAsAtomicUnit=on
  NtcPassd : Subsystem  TreatAsAtomicUnit=on
  NtcSts : Outport
  wires:
  StHlthErr/1 -> If/1
  If/1 -> NtcFaild/Action
  Merge/1 -> NtcSts/1
  NtcPassd/1(NtcPassd) -> Merge/2
  If/2 -> NtcPassd/Action
  NtcFaild/1(NtcFaild) -> Merge/1

== system ES105A_StHlthSigNormn/StHlthSigNormn/UpdRawSig/Motor Position 2 /NtcMotPosStHlth ==
  NtcNr : Inport
  NtcStInfo : Inport  Port=2
  NtcSts : Inport  Port=3
  DebStep : Inport  Port=4
  SetNtcSts : Subsystem  RequirementInfo={} %GIDa_e15acc41_e270_4229_a20a_2a1d705a48ba  TreatAsAtomicUnit=on
      settings: RTWSystemCode=Inline
  wires:
  NtcNr/1 -> SetNtcSts/1(NtcNr)  "NtcNr"
  NtcSts/1 -> SetNtcSts/3(NtcSts)
  DebStep/1 -> SetNtcSts/4(DebStep)
  NtcStInfo/1 -> SetNtcSts/2(NtcStInfo)

== system ES105A_StHlthSigNormn/StHlthSigNormn/UpdRawSig/Motor Position Error /AbsltMotPosABDifStHlth Calc ==
  MotAgABErrTerm : Inport
  Action Port : ActionPort  ActionType=case
  Constant : Constant  Value=StHlthSigNormnStHlthCorrlnErr
  CopyRight2 : Subsystem  Description=|  mask(Copyright Information){none=on}
      | Copyright info block.                                               
      |                                                                     
      | Place copyright information at the top of every subsystem in design.
      mask prompts: none "No parameters"
      mask help: Place copyright information at the top of every subsystem in design.
      mask Display:
      | NxtrConf = 'Nexteer Confidential';
      | 
      | sys = bdroot; %handle for the current model ("system")
      | first = get_param(sys,'Created');
      | first = first(end-3:end);  %year is last four digits
      | 
      | last = get_param(sys,'LastModifiedDate');
      | if isempty(last)
      |     last = datestr(now,'yyyy');
      | else
      |     last = last(end-3:end);
      | end
      | 
      | if strcmp(first,last)
      |     fprintf('%s -- Copyright %s Nexteer',NxtrConf,first)
      | else
      |     fprintf('%s -- %s%s- %s Nexteer',NxtrConf,char(169),first,last)
      | end
  If : If  IfExpression=u1
  If Action Subsystem : Subsystem  TreatAsAtomicUnit=on
  If Action Subsystem1 : Subsystem  TreatAsAtomicUnit=on
  LimStat_u2 : NxtrLim/LimStat_u08  LoLim=AbsltMotPosABDifStHlth.EngMin  HiLim=AbsltMotPosABDifStHlth.EngMax
      settings: AttributesFormatString=|
      | Low Limit: %<LoLim>
      | High Limit:%<HiLim>
  Merge : Merge
  Relational Operator : RelationalOperator  Operator=>  OutDataTypeStr=boolean
  AbsltMotPosABDifStHlth : Outport  InitialOutput=HLTH100PERC_CNT_U08
      settings: AttributesFormatString=Initial Output: %<InitialOutput>
  wires:
  MotAgABErrTerm/1 -> [MotAgABErrTerm], Relational Operator/1
  Constant/1 -> Relational Operator/2
  Relational Operator/1 -> If/1
  If/1 -> If Action Subsystem/Action
  If/2 -> If Action Subsystem1/Action
  [MotAgABErrTerm] -> If Action Subsystem/1(MotAgABErrTerm)
  If Action Subsystem/1(AbsltMotPosABDiffStHlth) -> Merge/1
  If Action Subsystem1/1(AbsltMotPosABDiffStHlth) -> Merge/2
  Merge/1 -> LimStat_u2/1
  LimStat_u2/1 -> AbsltMotPosABDifStHlth/1

== system ES105A_StHlthSigNormn/StHlthSigNormn/UpdRawSig/Motor Position Error /AbsltMotPosACDifStHlth Calc ==
  MotAgACErrTerm : Inport
  Action Port : ActionPort  ActionType=case
  Constant2 : Constant  Value=StHlthSigNormnStHlthCorrlnErr
  CopyRight2 : Subsystem  Description=|  mask(Copyright Information){none=on}
      | Copyright info block.                                               
      |                                                                     
      | Place copyright information at the top of every subsystem in design.
      mask prompts: none "No parameters"
      mask help: Place copyright information at the top of every subsystem in design.
      mask Display:
      | NxtrConf = 'Nexteer Confidential';
      | 
      | sys = bdroot; %handle for the current model ("system")
      | first = get_param(sys,'Created');
      | first = first(end-3:end);  %year is last four digits
      | 
      | last = get_param(sys,'LastModifiedDate');
      | if isempty(last)
      |     last = datestr(now,'yyyy');
      | else
      |     last = last(end-3:end);
      | end
      | 
      | if strcmp(first,last)
      |     fprintf('%s -- Copyright %s Nexteer',NxtrConf,first)
      | else
      |     fprintf('%s -- %s%s- %s Nexteer',NxtrConf,char(169),first,last)
      | end
  If Action Subsystem4 : Subsystem  TreatAsAtomicUnit=on
  If Action Subsystem5 : Subsystem  TreatAsAtomicUnit=on
  If2 : If  IfExpression=u1
  LimStat_u1 : NxtrLim/LimStat_u08  LoLim=AbsltMotPosACDifStHlth.EngMin  HiLim=AbsltMotPosACDifStHlth.EngMax
      settings: AttributesFormatString=|
      | Low Limit: %<LoLim>
      | High Limit:%<HiLim>
  Merge1 : Merge
  Relational Operator2 : RelationalOperator  Operator=>  OutDataTypeStr=boolean
  AbsltMotPosACDifStHlth : Outport  InitialOutput=HLTH100PERC_CNT_U08
      settings: AttributesFormatString=Initial Output: %<InitialOutput>
  wires:
  MotAgACErrTerm/1 -> [MotAgACErrTerm], Relational Operator2/1
  Constant2/1 -> Relational Operator2/2
  Relational Operator2/1 -> If2/1
  If2/1 -> If Action Subsystem4/Action
  If2/2 -> If Action Subsystem5/Action
  [MotAgACErrTerm] -> If Action Subsystem4/1(MotAgACErrTerm)
  If Action Subsystem4/1(AbsltMotPosACDiffStHlth) -> Merge1/1
  If Action Subsystem5/1(AbsltMotPosACDiffStHlth) -> Merge1/2
  Merge1/1 -> LimStat_u1/1
  LimStat_u1/1 -> AbsltMotPosACDifStHlth/1
